simulink model "ame532Project1_GimbalDynamicsModel_2023a"  (R2023a)
settings: Solver=ode4  StartTime=0.0  StopTime=60  FixedStep=0.01  RelTol=1e-3
model workspace (MAT data in the model file):
  theta : Simulink.Parameter (value not decoded)
undefined symbols (not defined in the file): a0_s2, a0_s3, a0_s4, a0_s5, AR_s2, AR_s3, AR_s4, AR_s5, area_s2, area_s3, area_s4, area_s5, c_s2, c_s3, c_s4, c_s5, CD0_s2, CD0_s3, CD0_s4, CD0_s5, CDa_s2, CDa_s3, CDa_s4, CDa_s5, CL0_s2, CL0_s3, CL0_s4, CL0_s5, CM0_s2, CM0_s3, CM0_s4, CM0_s5, CMa_s2, CMa_s3, CMa_s4, CMa_s5, e_s2, e_s3, e_s4, e_s5, earthRadius, elevator_sA, i_s2, i_s3, i_s4, i_s5, Jxx, Jxy, Jxz, Jyx, Jyy, Jyz, Jzx, Jzy, Jzz, leftaileron_sA, LL, MM, n_s2, n_s3 ... (+12)
libraries: simulink_extras x35, matrix_library x23, aerolibutil x7, aerolibfltsims x4, vrlib x3, aerolibtransform2 x2, slpidlib x2, simulink x2, sharedutil x1
(part 2 of 4)

== system ame532Project1_GimbalDynamicsModel_2023a/Gimbal Aircraft dynamic sim/measurement subsystem ==
  velocity in body frame : Inport
  Asin : Trigonometry  Operator=asin
  Atan2 : Trigonometry  Operator=atan2
  Demux : Demux  Outputs=3
  Demux1 : Demux  Outputs=3
  Display : Display
  Divide : Product  Inputs=*/  RndMeth=Zero  SaturateOnIntegerOverflow=on
  MATLAB Function : MATLAB Function  TreatAsAtomicUnit=on
  Mux : Mux  Inputs=3
  Radians to Degrees{,1..3} (4 alike) : simulink_extras/Transformations/Radians to Degrees
  v_inf alpha beta : Scope  NumInputPorts=3
  total speed : Outport
  alpha (AoA) : Outport  Port=2
  beta (side slip) : Outport  Port=3
  wires:
  MATLAB Function/1(magnitude) -> Divide/2, Mux/1, total speed/1, v_inf alpha beta/1
  velocity in body frame/1 -> MATLAB Function/1(velocity), Demux1/1, Demux/1
  Demux/3 -> Atan2/1
  Demux/1 -> Atan2/2
  Atan2/1 -> alpha (AoA)/1, Radians to Degrees2/1, Radians to Degrees/1
  Demux1/2 -> Divide/1
  Divide/1 -> Asin/1
  Asin/1 -> beta (side slip)/1, Radians to Degrees3/1, Radians to Degrees1/1
  Mux/1 -> Display/1
  Radians to Degrees/1 -> Mux/2
  Radians to Degrees1/1 -> Mux/3
  Radians to Degrees2/1 -> v_inf alpha beta/2
  Radians to Degrees3/1 -> v_inf alpha beta/3

== system ame532Project1_GimbalDynamicsModel_2023a/Gimbal Aircraft dynamic sim/rotational dynamics ==
  note: body rate acceleration
  J_matrix : Inport
  Initial w : Inport  Port=2
  moment in body : Inport  Port=3
  Cross Product : matrix_library/Cross Product
  Display4 : Display
  Display5 : Display
  Display6 : Display
  Invert 3x3 Matrix : aerolibutil/Invert  3x3 Matrix
  Matrix Multiply4 : Product  Multiplication=Matrix(*)
  Matrix Multiply5 : Product  Multiplication=Matrix(*)
  Sum : Sum  Inputs=|+-
  body rate : Integrator  InitialConditionSource=external  InitialCondition=[0 0 0]'
  omega_b : Outport
  wires:
  Cross Product/1 -> Sum/2, Display6/1
  Sum/1 -> Matrix Multiply4/2
  J_matrix/1 -> Matrix Multiply5/1, Invert 3x3 Matrix/1
  body rate/1 -> omega_b/1, Matrix Multiply5/2, Cross Product/1
  Matrix Multiply4/1 -> Display5/1, body rate/1
  Invert 3x3 Matrix/1 -> Matrix Multiply4/1, Display4/1
  Matrix Multiply5/1 -> Cross Product/2
  Initial w/1 -> body rate/2
  moment in body/1 -> Sum/1

== system ame532Project1_GimbalDynamicsModel_2023a/Gimbal Aircraft dynamic sim/translational dynamics ==
  note: counter gravity before needs to be accounted by a DCM
  note: velocity in body frame
  note: acceleration in body frame
  p : Inport
  q : Inport  Port=2
  r : Inport  Port=3
  ZYXDCM : Inport  Port=4
  external forces : Inport  Port=5
  intial velocity : Inport  Port=6
  Display{,1..4,8..9} (7 alike) : Display
  Integrator5 : Integrator  InitialConditionSource=external
  MATLAB Function10 : MATLAB Function  TreatAsAtomicUnit=on
  Manual Switch : ManualSwitch
  Matrix Multiply6 : Product  Multiplication=Matrix(*)
  Matrix Multiply7 : Product  Multiplication=Matrix(*)
  Scope : Scope
  Sum : Sum  Inputs=|++-
  gravity in N_frame : Constant  Value=[0 0 9.81]'
  gravity in N_frame1 : Constant  Value=[0 0 0]'
  weight : Gain  Gain=1/0.48
  velocity in body frame : Outport
  wires:
  MATLAB Function10/1(Cross_Product_Matrix) -> Matrix Multiply7/1, Display8/1
  Integrator5/1 -> velocity in body frame/1, Display1/1, Matrix Multiply7/2
  Sum/1 -> Display3/1, Scope/1, Integrator5/1
  Matrix Multiply6/1 -> Sum/2, Display2/1
  Matrix Multiply7/1 -> Sum/3, Display9/1
  ZYXDCM/1 -> Display/1, Matrix Multiply6/1
  q/1 -> MATLAB Function10/2(q)
  p/1 -> MATLAB Function10/1(p)
  r/1 -> MATLAB Function10/3(r)
  intial velocity/1 -> Integrator5/2
  external forces/1 -> weight/1
  weight/1 -> Sum/1, Display4/1
  gravity in N_frame1/1 -> Manual Switch/2
  gravity in N_frame/1 -> Manual Switch/1
  Manual Switch/1 -> Matrix Multiply6/2

== system ame532Project1_GimbalDynamicsModel_2023a/Gimbal system/Controller  ==
  GA_Desired : Inport
  GA_True : Inport  Port=2
  Inport : Inport  Port=3
  J_Gimbal : Inport  Port=4
  Constant1 : Constant  Commented=on  Value=2
  Demux : Demux  Commented=on  Outputs=3
  Demux1 : Demux  Commented=on  Outputs=3
  Demux2 : Demux  Outputs=3
  Derivative : Derivative  Commented=on
  Derivative1 : Derivative  Commented=on
  Divide : Product  Commented=on  Inputs=*/
  Mux : Mux  Inputs=3
  PID Controller : slpidlib/PID Controller  Controller=PID  Form=Parallel  TimeDomain=Continuous-time  UseExternalTs=off  SampleTime=-1  IntegratorMethod=Forward Euler  FilterMethod=Forward Euler  ControllerParametersSource=internal  P=0.00204661863973543  I=7.76312130056365e-05  UseKiTs=off  D=0.0129825008664916  N=2.05306665016805  UseFilter=on  TunerSelectOption=Transfer Function Based (PID Tuner App)  InitialConditionSource=internal  InitialConditionForIntegrator=0  InitialConditionForFilter=0  DifferentiatorICPrevScaledInput=0  ExternalReset=none  TrackingMode=off  Kt=1  LimitOutput=off  SatLimitsSource=internal  UpperSaturationLimit=inf  LowerSaturationLimit=-inf  LinearizeAsGain=on  AntiWindupMode=none  Kb=1  LimitIntegrator=off  UpperIntegratorSaturationLimit=inf  LowerIntegratorSaturationLimit=-inf  POutMin=[]  POutMax=[]  IOutMin=[]  IOutMax=[]  DOutMin=[]  DOutMax=[]  NOutMin=[]  NOutMax=[]  SumOutMin=[]  SumOutMax=[]  SaturationOutMin=[]  SaturationOutMax=[]  PParamMin=[]  PParamMax=[]  IParamMin=[]  IParamMax=[]  DParamMin=[]  DParamMax=[]  NParamMin=[]  NParamMax=[]  KbParamMin=[]  KbParamMax=[]  KtParamMin=[]  KtParamMax=[]  KbOutMin=[]  KbOutMax=[]  KtOutMin=[]  KtOutMax=[]  IntegratorOutMin=[]  IntegratorOutMax=[]  FilterOutMin=[]  FilterOutMax=[]  SumI1OutMin=[]  SumI1OutMax=[]  SumI2OutMin=[]  SumI2OutMax=[]  SumI3OutMin=[]  SumI3OutMax=[]  SumI4OutMin=[]  SumI4OutMax=[]  SumDOutMin=[]  SumDOutMax=[]  DifferentiatorOutMin=[]  DifferentiatorOutMax=[]  FilterDiffOutCoefMin=[]  FilterDiffOutCoefMax=[]  ReciprocalOutMin=[]  ReciprocalOutMax=[]  SumDenOutMin=[]  SumDenOutMax=[]  SumNumOutMin=[]  SumNumOutMax=[]  DivideOutMin=[]  DivideOutMax=[]  UdiffTsProdOutMin=[]  UdiffTsProdOutMax=[]  NTsProdOutMin=[]  NTsProdOutMax=[]  UintegralTsProdOutMin=[]  UintegralTsProdOutMax=[]  UngainTsProdOutMin=[]  UngainTsProdOutMax=[]  ClampingZeroOutDataTypeStr=Inherit: Inherit via back propagation  ClampingZeroOutMin=[]  ClampingZeroOutMax=[]  FilterDenConstantOutDataTypeStr=Inherit: Inherit via back propagation  FilterDenConstantOutMin=[]  FilterDenConstantOutMax=[]  PCopyOutDataTypeStr=Inherit: Inherit via back propagation  PCopyOutMin=[]  PCopyOutMax=[]  NCopyOutDataTypeStr=Inherit: Inherit via back propagation  NCopyOutMin=[]  NCopyOutMax=[]  IntegratorContinuousStateAttributes=''  IntegratorStateMustResolveToSignalObject=off  IntegratorRTWStateStorageClass=Auto  FilterContinuousStateAttributes=''  FilterStateMustResolveToSignalObject=off  FilterRTWStateStorageClass=Auto  ParallelPVariant=InternalParameters  IdealPVariant=Disabled  IVariant=InternalParameters  DVariant=InternalParameters  IntegratorVariant=Continuous  SatVariant=Disabled  AWVariant=Passthrough  PCopyVariant=Disabled  TRVariant=Disabled  FdbkBlocksVariant=Forward  IdealPFdbkVariant=Disabled  SatFdbkVariant=Disabled  DerivativeFilterVariant=ContFilter  NVariant=InternalParameters  NCopyVariant=Disabled  FilterICVariant=InternalICsFilter  IntegratorICVariant=InternalICs  ExternalResetVariant=Disabled  TRSumVariant=Passthrough  SumFdbkVariant=Disabled  SumVariant=Sum_PID  TsampFilterVariant=InternalTs  TsampNgainVariant=Passthrough  TsampIntegralVariant=Disabled_SignalSpec  ExternalSaturationOutDataTypeStr=Inherit: Same as second input
  PID Controller1 : slpidlib/PID Controller  Controller=PID  Form=Parallel  TimeDomain=Continuous-time  UseExternalTs=off  SampleTime=-1  IntegratorMethod=Forward Euler  FilterMethod=Forward Euler  ControllerParametersSource=internal  P=-0.109538604051299  I=-0.0257010089513843  UseKiTs=off  D=-0.114637714712046  N=27.3346026399604  UseFilter=on  TunerSelectOption=Transfer Function Based (PID Tuner App)  InitialConditionSource=internal  InitialConditionForIntegrator=0  InitialConditionForFilter=0  DifferentiatorICPrevScaledInput=0  ExternalReset=none  TrackingMode=off  Kt=1  LimitOutput=off  SatLimitsSource=internal  UpperSaturationLimit=inf  LowerSaturationLimit=-inf  LinearizeAsGain=on  AntiWindupMode=none  Kb=1  LimitIntegrator=off  UpperIntegratorSaturationLimit=inf  LowerIntegratorSaturationLimit=-inf  POutMin=[]  POutMax=[]  IOutMin=[]  IOutMax=[]  DOutMin=[]  DOutMax=[]  NOutMin=[]  NOutMax=[]  SumOutMin=[]  SumOutMax=[]  SaturationOutMin=[]  SaturationOutMax=[]  PParamMin=[]  PParamMax=[]  IParamMin=[]  IParamMax=[]  DParamMin=[]  DParamMax=[]  NParamMin=[]  NParamMax=[]  KbParamMin=[]  KbParamMax=[]  KtParamMin=[]  KtParamMax=[]  KbOutMin=[]  KbOutMax=[]  KtOutMin=[]  KtOutMax=[]  IntegratorOutMin=[]  IntegratorOutMax=[]  FilterOutMin=[]  FilterOutMax=[]  SumI1OutMin=[]  SumI1OutMax=[]  SumI2OutMin=[]  SumI2OutMax=[]  SumI3OutMin=[]  SumI3OutMax=[]  SumI4OutMin=[]  SumI4OutMax=[]  SumDOutMin=[]  SumDOutMax=[]  DifferentiatorOutMin=[]  DifferentiatorOutMax=[]  FilterDiffOutCoefMin=[]  FilterDiffOutCoefMax=[]  ReciprocalOutMin=[]  ReciprocalOutMax=[]  SumDenOutMin=[]  SumDenOutMax=[]  SumNumOutMin=[]  SumNumOutMax=[]  DivideOutMin=[]  DivideOutMax=[]  UdiffTsProdOutMin=[]  UdiffTsProdOutMax=[]  NTsProdOutMin=[]  NTsProdOutMax=[]  UintegralTsProdOutMin=[]  UintegralTsProdOutMax=[]  UngainTsProdOutMin=[]  UngainTsProdOutMax=[]  ClampingZeroOutDataTypeStr=Inherit: Inherit via back propagation  ClampingZeroOutMin=[]  ClampingZeroOutMax=[]  FilterDenConstantOutDataTypeStr=Inherit: Inherit via back propagation  FilterDenConstantOutMin=[]  FilterDenConstantOutMax=[]  PCopyOutDataTypeStr=Inherit: Inherit via back propagation  PCopyOutMin=[]  PCopyOutMax=[]  NCopyOutDataTypeStr=Inherit: Inherit via back propagation  NCopyOutMin=[]  NCopyOutMax=[]  IntegratorContinuousStateAttributes=''  IntegratorStateMustResolveToSignalObject=off  IntegratorRTWStateStorageClass=Auto  FilterContinuousStateAttributes=''  FilterStateMustResolveToSignalObject=off  FilterRTWStateStorageClass=Auto  ParallelPVariant=InternalParameters  IdealPVariant=Disabled  IVariant=InternalParameters  DVariant=InternalParameters  IntegratorVariant=Continuous  SatVariant=Disabled  AWVariant=Passthrough  PCopyVariant=Disabled  TRVariant=Disabled  FdbkBlocksVariant=Forward  IdealPFdbkVariant=Disabled  SatFdbkVariant=Disabled  DerivativeFilterVariant=ContFilter  NVariant=InternalParameters  NCopyVariant=Disabled  FilterICVariant=InternalICsFilter  IntegratorICVariant=InternalICs  ExternalResetVariant=Disabled  TRSumVariant=Passthrough  SumFdbkVariant=Disabled  SumVariant=Sum_PID  TsampFilterVariant=InternalTs  TsampNgainVariant=Passthrough  TsampIntegralVariant=Disabled_SignalSpec  ExternalSaturationOutDataTypeStr=Inherit: Same as second input
  Product : Product  Commented=on
  Product1 : Product  Commented=on
  Product2 : Product  Multiplication=Matrix(*)
  Scope : Scope
  Scope1 : Scope
  Square : Math  Commented=on  Operator=square
  Subtract : Sum  Inputs=+-
  Subtract1 : Sum  Commented=on  Inputs=+-
  time : Constant  Commented=on  Value=5
  Torque_Cmd : Outport
  wires:
  GA_Desired/1 -> Subtract/1
  GA_True/1 -> Subtract/2
  Derivative/1 -> Derivative1/1
  Derivative1/1 -> Demux1/1
  Inport/1 -> Product/1
  time/1 -> Product/2, Square/1
  Product/1 -> Subtract1/2
  Subtract1/1 -> Product1/1
  Constant1/1 -> Product1/2
  Product1/1 -> Divide/1
  Square/1 -> Divide/2
  Product2/1 -> Scope1/1
  Subtract/1 -> Demux2/1
  Demux2/2 -> PID Controller/1
  Demux2/3 -> PID Controller1/1
  PID Controller/1 -> Mux/2
  PID Controller1/1 -> Mux/3
  Demux2/1 -> Mux/1
  Mux/1 -> Torque_Cmd/1

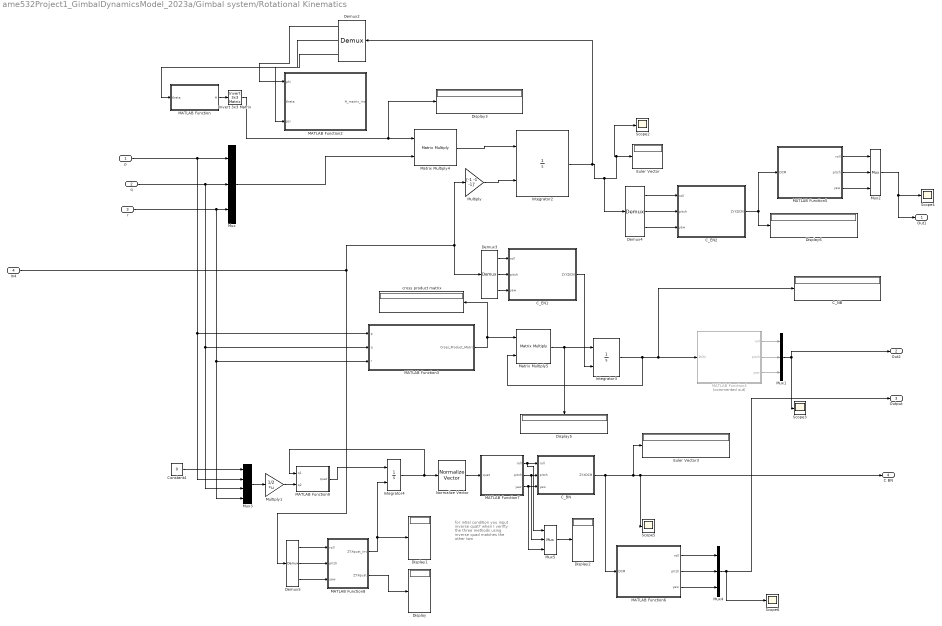
== system ame532Project1_GimbalDynamicsModel_2023a/Gimbal system/Rotational Kinematics ==
  note: for intial condition you input inverse quat?
      | when I verifty the three methods using inverse quad matches the other two
  p : Inport
  q : Inport  Port=2
  r : Inport  Port=3
  In4 : Inport  Port=4
  C_BN : MATLAB Function  TreatAsAtomicUnit=on
  C_EN1 : MATLAB Function  TreatAsAtomicUnit=on
  C_EN2 : MATLAB Function  TreatAsAtomicUnit=on
  C_NB : Display
  Constant4 : Constant  Value=0
  Demux{2..5} (4 alike) : Demux  Outputs=3
  Display{,1..3,5..6} (6 alike) : Display
  Euler Vector : Display
  Euler Vector3 : Display
  Integrator2 : Integrator  InitialConditionSource=external
  Integrator3 : Integrator  InitialConditionSource=external
  Integrator4 : Integrator  InitialConditionSource=external  InitialCondition=[1 0 0 0]'
  Invert 3x3 Matrix : aerolibutil/Invert  3x3 Matrix
  MATLAB Function : MATLAB Function  TreatAsAtomicUnit=on
  MATLAB Function2 : MATLAB Function  TreatAsAtomicUnit=on
  MATLAB Function3 : MATLAB Function  TreatAsAtomicUnit=on
  MATLAB Function4 : MATLAB Function  Commented=on  TreatAsAtomicUnit=on
  MATLAB Function5 : MATLAB Function  TreatAsAtomicUnit=on
  MATLAB Function6 : MATLAB Function  TreatAsAtomicUnit=on
  MATLAB Function7 : MATLAB Function  TreatAsAtomicUnit=on
  MATLAB Function8 : MATLAB Function  TreatAsAtomicUnit=on
  MATLAB Function9 : MATLAB Function  TreatAsAtomicUnit=on
  Matrix Multiply4 : Product  Multiplication=Matrix(*)
  Matrix Multiply5 : Product  Multiplication=Matrix(*)
  Multiply : Gain  Gain=[-1 -1 -1]'
  Multiply1 : Gain  Gain=1/2  Multiplication=Matrix(K*u)
  Mux{,1..2,4..5} (5 alike) : Mux  Inputs=3
  Mux3 : Mux
  Normalize Vector : vrlib/Utilities/Normalize Vector  maxzero=0
  Scope{2..6} (5 alike) : Scope
  cross product matrix : Display
  Out1 : Outport
  Out2 : Outport  Port=2
  Output : Outport  Port=3
  C BN : Outport  Port=4
  wires:
  Matrix Multiply4/1 -> Integrator2/1
  In4/1 -> Multiply/1, Demux3/1, Demux5/1
  MATLAB Function4/3(yaw) -> Mux1/3
  Integrator2/1 -> Scope2/1, Euler Vector/1, Demux4/1, Demux2/1
  MATLAB Function6/2(pitch) -> Mux4/2
  r/1 -> Mux3/4, MATLAB Function3/3(r), Mux/3
  Matrix Multiply5/1 -> Display5/1, Integrator3/1
  Mux/1 -> Matrix Multiply4/2
  q/1 -> Mux3/3, MATLAB Function3/2(q), Mux/2
  C_BN/1(ZYXDCM) -> MATLAB Function6/1(DCM), C BN/1, Scope5/1, Euler Vector3/1
  C_EN1/1(ZYXDCM) -> Integrator3/2
  MATLAB Function5/2(pitch) -> Mux2/2
  Mux1/1 -> Out2/1, Scope3/1
  MATLAB Function4/1(roll) -> Mux1/1
  Demux2/2 -> MATLAB Function/1(theta)
  Demux4/3 -> C_EN2/3(yaw)
  MATLAB Function4/2(pitch) -> Mux1/2
  Demux2/3 -> MATLAB Function2/3(psi)
  Demux2/1 -> MATLAB Function2/1(phi)
  Demux5/1 -> MATLAB Function8/1(roll)
  Demux3/1 -> C_EN1/1(roll)
  Demux5/2 -> MATLAB Function8/2(pitch)
  Demux4/1 -> C_EN2/1(roll)
  Demux3/3 -> C_EN1/3(yaw)
  Multiply/1 -> Integrator2/2
  C_EN2/1(ZYXDCM) -> Display6/1, MATLAB Function5/1(DCM)
  Normalize Vector/1 -> MATLAB Function7/1(quat)
  MATLAB Function9/1(quat) -> Integrator4/1
  Integrator3/1 -> Matrix Multiply5/2, MATLAB Function4/1(DCM), C_NB/1
  p/1 -> Mux3/2, MATLAB Function3/1(p), Mux/1
  Integrator4/1 -> Normalize Vector/1, MATLAB Function9/1(q1)
  MATLAB Function7/3(yaw) -> Mux5/3, C_BN/3(yaw)
  Mux2/1 -> Out1/1, Scope4/1
  MATLAB Function5/3(yaw) -> Mux2/3
  Constant4/1 -> Mux3/1
  Mux3/1 -> Multiply1/1
  Mux4/1 -> Output/1, Scope6/1
  MATLAB Function7/1(roll) -> Mux5/1, C_BN/1(roll)
  MATLAB Function5/1(roll) -> Mux2/1
  Demux5/3 -> MATLAB Function8/3(yaw)
  MATLAB Function6/1(roll) -> Mux4/1
  MATLAB Function6/3(yaw) -> Mux4/3
  Multiply1/1 -> MATLAB Function9/2(q2)
  MATLAB Function3/1(Cross_Product_Matrix) -> Matrix Multiply5/1, cross product matrix/1
  Demux4/2 -> C_EN2/2(pitch)
  Demux3/2 -> C_EN1/2(pitch)
  MATLAB Function7/2(pitch) -> Mux5/2, C_BN/2(pitch)
  MATLAB Function8/1(ZYXquat_inv) -> Integrator4/2, Display1/1
  MATLAB Function8/2(ZYXquat) -> Display/1
  Mux5/1 -> Display2/1
  MATLAB Function/1(H) -> Invert 3x3 Matrix/1
  Invert 3x3 Matrix/1 -> Display3/1, Matrix Multiply4/1

== system ame532Project1_GimbalDynamicsModel_2023a/Gimbal system/rotational dynamics gimbal ==
  note: body acceleration
  J_matrix : Inport
  Initial w : Inport  Port=2
  Tcmd : Inport  Port=3
  Cross Product : matrix_library/Cross Product
  Display4 : Display
  Display5 : Display
  Display6 : Display
  Invert 3x3 Matrix : aerolibutil/Invert  3x3 Matrix
  Matrix Multiply4 : Product  Multiplication=Matrix(*)
  Matrix Multiply5 : Product  Multiplication=Matrix(*)
  Sum : Sum  Inputs=|+-
  body rate : Integrator  InitialConditionSource=external  InitialCondition=[0 0 0]'
  w_b : Outport
  Outport : Outport  Port=2
  wires:
  Cross Product/1 -> Sum/2, Display6/1
  Sum/1 -> Matrix Multiply4/2
  J_matrix/1 -> Matrix Multiply5/1, Invert 3x3 Matrix/1
  body rate/1 -> w_b/1, Matrix Multiply5/2, Cross Product/1
  Matrix Multiply4/1 -> Display5/1, Outport/1, body rate/1
  Matrix Multiply5/1 -> Cross Product/2
  Initial w/1 -> body rate/2
  Tcmd/1 -> Sum/1
  Invert 3x3 Matrix/1 -> Display4/1, Matrix Multiply4/1

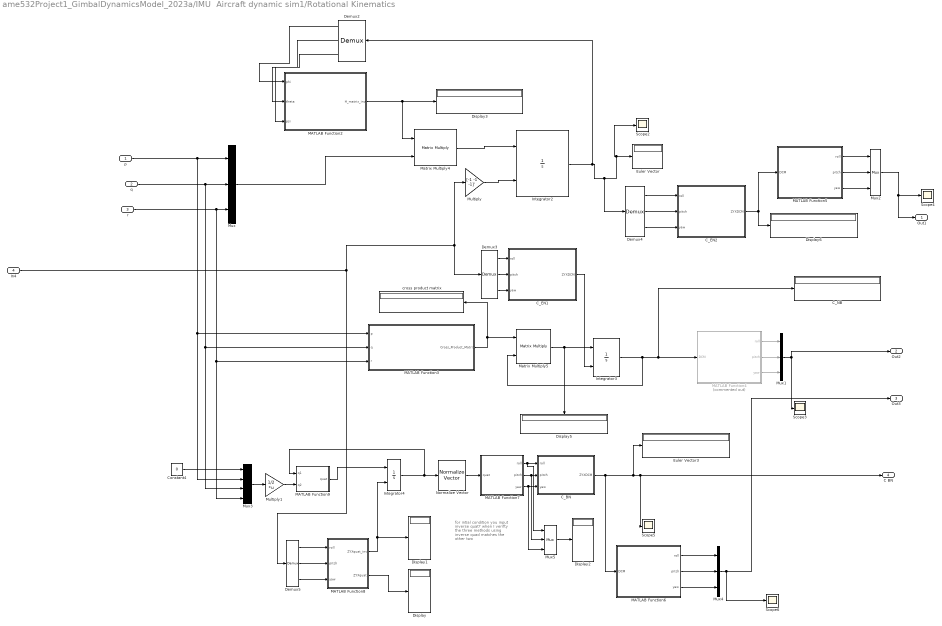
== system ame532Project1_GimbalDynamicsModel_2023a/IMU  Aircraft dynamic sim1/Rotational Kinematics ==
  note: for intial condition you input inverse quat?
      | when I verifty the three methods using inverse quad matches the other two
  p : Inport
  q : Inport  Port=2
  r : Inport  Port=3
  In4 : Inport  Port=4
  C_BN : MATLAB Function  TreatAsAtomicUnit=on
  C_EN1 : MATLAB Function  TreatAsAtomicUnit=on
  C_EN2 : MATLAB Function  TreatAsAtomicUnit=on
  C_NB : Display
  Constant4 : Constant  Value=0
  Demux{2..5} (4 alike) : Demux  Outputs=3
  Display{,1..3,5..6} (6 alike) : Display
  Euler Vector : Display
  Euler Vector3 : Display
  Integrator2 : Integrator  InitialConditionSource=external
  Integrator3 : Integrator  InitialConditionSource=external
  Integrator4 : Integrator  InitialConditionSource=external  InitialCondition=[1 0 0 0]'
  MATLAB Function2 : MATLAB Function  TreatAsAtomicUnit=on
  MATLAB Function3 : MATLAB Function  TreatAsAtomicUnit=on
  MATLAB Function4 : MATLAB Function  Commented=on  TreatAsAtomicUnit=on
  MATLAB Function5 : MATLAB Function  TreatAsAtomicUnit=on
  MATLAB Function6 : MATLAB Function  TreatAsAtomicUnit=on
  MATLAB Function7 : MATLAB Function  TreatAsAtomicUnit=on
  MATLAB Function8 : MATLAB Function  TreatAsAtomicUnit=on
  MATLAB Function9 : MATLAB Function  TreatAsAtomicUnit=on
  Matrix Multiply4 : Product  Multiplication=Matrix(*)
  Matrix Multiply5 : Product  Multiplication=Matrix(*)
  Multiply : Gain  Gain=[-1 -1 -1]'
  Multiply1 : Gain  Gain=1/2  Multiplication=Matrix(K*u)
  Mux{,1..2,4..5} (5 alike) : Mux  Inputs=3
  Mux3 : Mux
  Normalize Vector : vrlib/Utilities/Normalize Vector  maxzero=0
  Scope{2..6} (5 alike) : Scope
  cross product matrix : Display
  Out1 : Outport
  Out2 : Outport  Port=2
  Out3 : Outport  Port=3
  C BN : Outport  Port=4
  wires:
  Matrix Multiply4/1 -> Integrator2/1
  In4/1 -> Multiply/1, Demux3/1, Demux5/1
  MATLAB Function4/3(yaw) -> Mux1/3
  Integrator2/1 -> Scope2/1, Euler Vector/1, Demux4/1, Demux2/1
  MATLAB Function2/1(H_matrix_inv) -> Display3/1, Matrix Multiply4/1
  MATLAB Function6/2(pitch) -> Mux4/2
  r/1 -> Mux3/4, MATLAB Function3/3(r), Mux/3
  Matrix Multiply5/1 -> Display5/1, Integrator3/1
  Mux/1 -> Matrix Multiply4/2
  q/1 -> Mux3/3, MATLAB Function3/2(q), Mux/2
  C_BN/1(ZYXDCM) -> MATLAB Function6/1(DCM), C BN/1, Scope5/1, Euler Vector3/1
  C_EN1/1(ZYXDCM) -> Integrator3/2
  MATLAB Function5/2(pitch) -> Mux2/2
  Mux1/1 -> Out2/1, Scope3/1
  MATLAB Function4/1(roll) -> Mux1/1
  Demux2/2 -> MATLAB Function2/2(theta)
  Demux4/3 -> C_EN2/3(yaw)
  MATLAB Function4/2(pitch) -> Mux1/2
  Demux2/3 -> MATLAB Function2/3(psi)
  Demux2/1 -> MATLAB Function2/1(phi)
  Demux5/1 -> MATLAB Function8/1(roll)
  Demux3/1 -> C_EN1/1(roll)
  Demux5/2 -> MATLAB Function8/2(pitch)
  Demux4/1 -> C_EN2/1(roll)
  Demux3/3 -> C_EN1/3(yaw)
  Multiply/1 -> Integrator2/2
  C_EN2/1(ZYXDCM) -> Display6/1, MATLAB Function5/1(DCM)
  Normalize Vector/1 -> MATLAB Function7/1(quat)
  MATLAB Function9/1(quat) -> Integrator4/1
  Integrator3/1 -> Matrix Multiply5/2, MATLAB Function4/1(DCM), C_NB/1
  p/1 -> Mux3/2, MATLAB Function3/1(p), Mux/1
  Integrator4/1 -> Normalize Vector/1, MATLAB Function9/1(q1)
  MATLAB Function7/3(yaw) -> Mux5/3, C_BN/3(yaw)
  Mux2/1 -> Out1/1, Scope4/1
  MATLAB Function5/3(yaw) -> Mux2/3
  Constant4/1 -> Mux3/1
  Mux3/1 -> Multiply1/1
  Mux4/1 -> Out3/1, Scope6/1
  MATLAB Function7/1(roll) -> Mux5/1, C_BN/1(roll)
  MATLAB Function5/1(roll) -> Mux2/1
  Demux5/3 -> MATLAB Function8/3(yaw)
  MATLAB Function6/1(roll) -> Mux4/1
  MATLAB Function6/3(yaw) -> Mux4/3
  Multiply1/1 -> MATLAB Function9/2(q2)
  MATLAB Function3/1(Cross_Product_Matrix) -> Matrix Multiply5/1, cross product matrix/1
  Demux4/2 -> C_EN2/2(pitch)
  Demux3/2 -> C_EN1/2(pitch)
  MATLAB Function7/2(pitch) -> Mux5/2, C_BN/2(pitch)
  MATLAB Function8/1(ZYXquat_inv) -> Integrator4/2, Display1/1
  MATLAB Function8/2(ZYXquat) -> Display/1
  Mux5/1 -> Display2/1

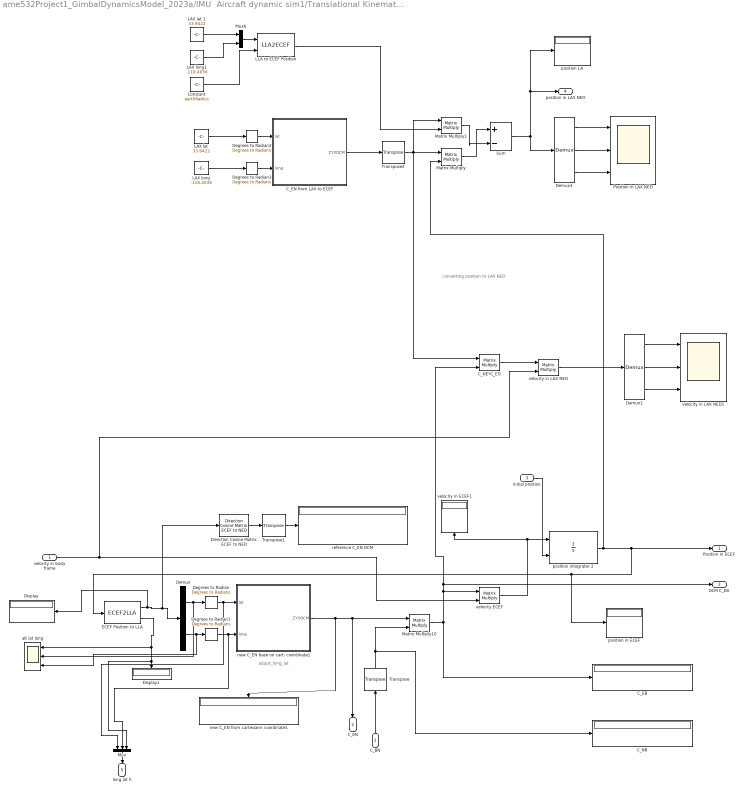
== system ame532Project1_GimbalDynamicsModel_2023a/IMU  Aircraft dynamic sim1/Translational Kinematics ==
  note: converting position to LAX NED
  note: adjust_long_lat
  velocity in body frame : Inport
  C_BN : Inport  Port=2
  initial position : Inport  Port=3
  C_EB : Display
  C_EN from LAX to ECEF : MATLAB Function  TreatAsAtomicUnit=on
  C_NB : Display
  C_NE*C_EO : Product  Multiplication=Matrix(*)
  Constant : Constant  Value=earthRadius
  Degrees to Radian{,1..3} (4 alike) : simulink_extras/Transformations/Degrees to Radians
  Demux : Demux  Outputs=2
  Demux1 : Demux  Outputs=3
  Demux3 : Demux  Outputs=3
  Direction Cosine Matrix ECEF to NED : aerolibtransform2/Direction Cosine Matrix ECEF to NED
  Display : Display
  Display1 : Display
  ECEF Position to LLA : ECEF2LLA  ptype=Custom  R=earthRadius
  "LAX lat " : Constant  Value=33.9422
  LAX lat 1 : Constant  Value=33.9422
  LAX long : Constant  Value=-118.4036
  LAX long1 : Constant  Value=-118.4036
  LLA to ECEF Position : LLA2ECEF
  Matrix Multiply : Product  Multiplication=Matrix(*)
  Matrix Multiply1 : Product  Multiplication=Matrix(*)
  Matrix Multiply10 : Product  Multiplication=Matrix(*)
  Mux : Mux  Inputs=3
  Mux6 : Mux  Inputs=2
  Position in LAX NED : Scope  NumInputPorts=3
  Sum : Sum  Inputs=|+-
  Transpose : matrix_library/Transpose
  Transpose1 : matrix_library/Transpose
  Transpose2 : matrix_library/Transpose
  alt lat long : Scope  NumInputPorts=3
  new C_EN base on cart. coordinate1 : MATLAB Function  TreatAsAtomicUnit=on
  new C_EN from cartesiann coordinate1 : Display
  "position LA " : Display
  position in ECEF : Display
  position integrator 2 : Integrator  InitialConditionSource=external  InitialCondition=[6378100,0,0]'
  reference C_EN DCM : Display
  velocity ECEF : Product  Multiplication=Matrix(*)
  velocity in ECEF1 : Display
  velocity in LAX NED : Product  Multiplication=Matrix(*)
  velocity in LAX NED1 : Scope  NumInputPorts=3
  Position in ECEF : Outport
  C_EN : Outport  Port=2
  DCM C_EB : Outport  Port=3
  position in LAX NED : Outport  Port=4
  long lat h : Outport  Port=5
  wires:
  initial position/1 -> position integrator 2/2
  new C_EN base on cart. coordinate1/1(ZYXDCM) -> new C_EN from cartesiann coordinate1/1, C_EN/1, Matrix Multiply10/1
  Matrix Multiply10/1 -> C_EB/1, DCM C_EB/1, C_NE*C_EO/2, velocity ECEF/1
  velocity ECEF/1 -> position integrator 2/1, velocity in ECEF1/1
  velocity in body frame/1 -> velocity in LAX NED/2, velocity ECEF/2
  C_BN/1 -> Transpose/1
  ECEF Position to LLA/1 -> Direction Cosine Matrix ECEF to NED/1, Demux/1, Display/1
  ECEF Position to LLA/2 -> alt lat long/1, Mux/3, Display1/1
  Demux/1 -> Degrees to Radian/1, alt lat long/2
  Demux/2 -> alt lat long/3, Degrees to Radian1/1
  Degrees to Radian/1 -> Mux/1, new C_EN base on cart. coordinate1/1(lat)
  Degrees to Radian1/1 -> Mux/2, new C_EN base on cart. coordinate1/2(long)
  Transpose/1 -> C_NB/1, Matrix Multiply10/2
  Direction Cosine Matrix ECEF to NED/1 -> Transpose1/1
  Transpose1/1 -> reference C_EN DCM/1
  Mux/1 -> long lat h/1
  "LAX lat "/1 -> Degrees to Radian2/1
  LAX long/1 -> Degrees to Radian3/1
  Degrees to Radian2/1 -> C_EN from LAX to ECEF/1(lat)
  Degrees to Radian3/1 -> C_EN from LAX to ECEF/2(long)
  C_EN from LAX to ECEF/1(ZYXDCM) -> Transpose2/1
  Demux3/2 -> Position in LAX NED/2
  Demux3/3 -> Position in LAX NED/3
  Demux3/1 -> Position in LAX NED/1
  Transpose2/1 -> C_NE*C_EO/1, Matrix Multiply1/1, Matrix Multiply/1
  LAX long1/1 -> Mux6/2
  LAX lat 1/1 -> Mux6/1
  Constant/1 -> LLA to ECEF Position/2
  Mux6/1 -> LLA to ECEF Position/1
  LLA to ECEF Position/1 -> Matrix Multiply1/2
  Matrix Multiply/1 -> Sum/1
  Matrix Multiply1/1 -> Sum/2
  Sum/1 -> "position LA "/1, position in LAX NED/1, Demux3/1
  position integrator 2/1 -> Position in ECEF/1, ECEF Position to LLA/1, position in ECEF/1, Matrix Multiply/2
  C_NE*C_EO/1 -> velocity in LAX NED/1
  Demux1/2 -> velocity in LAX NED1/2
  velocity in LAX NED/1 -> Demux1/1
  Demux1/3 -> velocity in LAX NED1/3
  Demux1/1 -> velocity in LAX NED1/1

== system ame532Project1_GimbalDynamicsModel_2023a/IMU  Aircraft dynamic sim1/Unused tranlational kinmatics ==
  In1 : Inport
  In2 : Inport  Port=2
  In3 : Inport  Port=3
  C_EN4 : MATLAB Function  TreatAsAtomicUnit=on
  DCM4 : Display
  Matrix Multiply8 : Product  Multiplication=Matrix(*)
  Matrix Multiply9 : Product  Multiplication=Matrix(*)
  Scope7 : Scope
  Transpose : matrix_library/Transpose
  pitch4 : Constant  Value=pi/2
  position integrator 1 : Integrator  InitialConditionSource=external  InitialCondition=[6378100,0,0]'
  position vector2 : Display
  roll4 : Constant  Value=0
  velocity in earth frame : Display
  yaw4 : Constant  Value=0
  wires:
  Matrix Multiply9/1 -> DCM4/1, Matrix Multiply8/1
  position integrator 1/1 -> Scope7/1, position vector2/1
  C_EN4/1(ZYXDCM) -> Matrix Multiply9/1
  Matrix Multiply8/1 -> velocity in earth frame/1, position integrator 1/1
  yaw4/1 -> C_EN4/3(yaw)
  pitch4/1 -> C_EN4/2(pitch)
  Transpose/1 -> Matrix Multiply9/2
  roll4/1 -> C_EN4/1(roll)
  In2/1 -> Matrix Multiply8/2
  In1/1 -> position integrator 1/2
  In3/1 -> Transpose/1

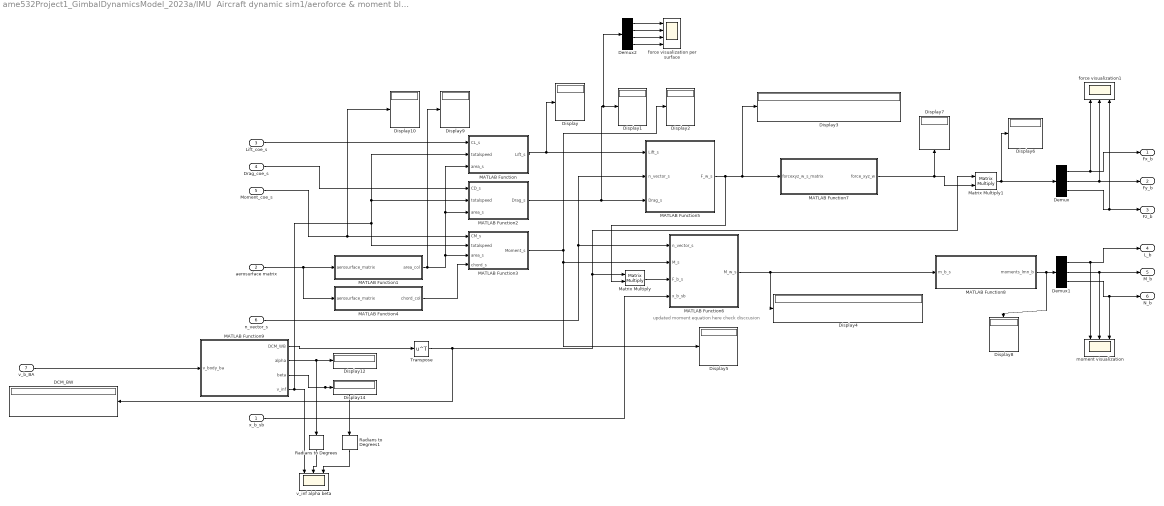
== system ame532Project1_GimbalDynamicsModel_2023a/IMU  Aircraft dynamic sim1/aeroforce & moment block ==
  note: updated moment equation here check disccusion
  x_b_sb : Inport
  aerosurface matrix : Inport  Port=2
  Lift_coe_s : Inport  Port=3
  Drag_coe_s : Inport  Port=4
  Moment_coe_s : Inport  Port=5
  n_vector_s : Inport  Port=6
  v_b_BA : Inport  Port=7
  DCM_BW : Display
  Demux : Demux  Outputs=3
  Demux1 : Demux  Outputs=3
  Demux2 : Demux
  Display{,1..10,12,14} (13 alike) : Display
  MATLAB Function : MATLAB Function  TreatAsAtomicUnit=on
  MATLAB Function1 : MATLAB Function  TreatAsAtomicUnit=on
  MATLAB Function2 : MATLAB Function  TreatAsAtomicUnit=on
  MATLAB Function3 : MATLAB Function  TreatAsAtomicUnit=on
  MATLAB Function4 : MATLAB Function  TreatAsAtomicUnit=on
  MATLAB Function5 : MATLAB Function  TreatAsAtomicUnit=on
  MATLAB Function6 : MATLAB Function  TreatAsAtomicUnit=on
  MATLAB Function7 : MATLAB Function  TreatAsAtomicUnit=on
  MATLAB Function8 : MATLAB Function  TreatAsAtomicUnit=on
  MATLAB Function9 : MATLAB Function  TreatAsAtomicUnit=on
  Matrix Multiply : Product  Multiplication=Matrix(*)
  Matrix Multiply1 : Product  Multiplication=Matrix(*)
  Radians to Degrees : simulink_extras/Transformations/Radians to Degrees
  Radians to Degrees1 : simulink_extras/Transformations/Radians to Degrees
  Transpose : Math  Operator=transpose
  force visualization per surface : Scope  NumInputPorts=4
  force visualization1 : Scope  NumInputPorts=3
  moment visualization : Scope  NumInputPorts=3
  v_inf alpha beta : Scope  NumInputPorts=3
  Fx_b : Outport
  Fy_b : Outport  Port=2
  Fz_b : Outport  Port=3
  L_b : Outport  Port=4
  M_b : Outport  Port=5
  N_b : Outport  Port=6
  wires:
  Lift_coe_s/1 -> MATLAB Function/1(CL_s)
  MATLAB Function9/4(v_inf) -> v_inf alpha beta/1, MATLAB Function2/2(totalspeed), MATLAB Function/2(totalspeed), MATLAB Function3/2(totalspeed)
  aerosurface matrix/1 -> MATLAB Function4/1(aerosurface_matrix), MATLAB Function1/1(aerosurface_matrix)
  MATLAB Function1/1(area_col) -> Display9/1, MATLAB Function2/3(area_s), MATLAB Function/3(area_s), MATLAB Function3/3(area_s)
  Drag_coe_s/1 -> MATLAB Function2/1(CD_s)
  Moment_coe_s/1 -> Display10/1, MATLAB Function3/1(CM_s)
  MATLAB Function4/1(chord_col) -> MATLAB Function3/4(chord_s)
  n_vector_s/1 -> MATLAB Function5/2(n_vector_s), MATLAB Function6/1(n_vector_s)
  MATLAB Function/1(Lift_s) -> Display/1, MATLAB Function5/1(Lift_s)
  MATLAB Function2/1(Drag_s) -> MATLAB Function5/3(Drag_s), Demux2/1, Display1/1
  MATLAB Function3/1(Moment_s) -> Display5/1, MATLAB Function6/2(M_s), Display2/1
  MATLAB Function6/1(M_w_s) -> Display4/1, MATLAB Function8/1(m_b_s)
  Matrix Multiply/1 -> MATLAB Function6/3(F_b_s)
  x_b_sb/1 -> MATLAB Function6/4(x_b_sb)
  MATLAB Function5/1(F_w_s) -> Matrix Multiply/2, Display3/1, MATLAB Function7/1(forcexyz_w_s_matrix)
  MATLAB Function7/1(force_xyz_w) -> Matrix Multiply1/2, Display7/1
  MATLAB Function8/1(moments_lmn_b) -> Demux1/1, Display8/1
  Matrix Multiply1/1 -> Demux/1, Display6/1
  MATLAB Function9/1(DCM_WB) -> Transpose/1
  v_b_BA/1 -> MATLAB Function9/1(v_body_ba)
  MATLAB Function9/2(alpha) -> Radians to Degrees/1, Display12/1
  MATLAB Function9/3(beta) -> Display14/1, Radians to Degrees1/1
  Demux1/1 -> L_b/1, moment visualization/1
  Demux1/2 -> M_b/1, moment visualization/2
  Demux1/3 -> moment visualization/3, N_b/1
  Demux/1 -> Fx_b/1, force visualization1/1
  Demux/2 -> Fy_b/1, force visualization1/2
  Demux/3 -> Fz_b/1, force visualization1/3
  Transpose/1 -> Matrix Multiply1/1, Matrix Multiply/1, DCM_BW/1
  Radians to Degrees/1 -> v_inf alpha beta/2
  Radians to Degrees1/1 -> v_inf alpha beta/3
  Demux2/4 -> force visualization per surface/4
  Demux2/3 -> force visualization per surface/3
  Demux2/2 -> force visualization per surface/2
  Demux2/1 -> force visualization per surface/1

== system ame532Project1_GimbalDynamicsModel_2023a/IMU  Aircraft dynamic sim1/aeroforce coefficient block ==
  note: next step is to create lift force, CD, CM
  aero surface property matrix : Inport
  real wind in N axes : Inport  Port=2
  velocity in bodyframe : Inport  Port=3
  C_BN : Inport  Port=4
  CD0 : Constant  Value=[0.01 0.01 0.01 0.01]'
  CD1 : Constant  Value=[0.9 0.9 0.8 0.8]'
  CD_a : Constant  Value=[1 1 1 1]'
  CL over time : Scope  NumInputPorts=4
  CL0 : Constant  Value=[0.05 0.05 0 0]'
  CM_0 : Constant  Value=[-0.05 -0.05 0 0]'
  CM_a : Constant  Value=[0 0 0 0]'
  Demux1 : Demux
  Demux5 : Demux
  Demux6 : Demux  Outputs=3
  Display{,1..3,5..7} (7 alike) : Display
  MATLAB Function : MATLAB Function  TreatAsAtomicUnit=on
  MATLAB Function1 : MATLAB Function  TreatAsAtomicUnit=on
  MATLAB Function2 : MATLAB Function  TreatAsAtomicUnit=on
  MATLAB Function3 : MATLAB Function  TreatAsAtomicUnit=on
  alpha : Scope  NumInputPorts=4
  alpha_0 : Constant  Value=[0.05 0.05 0 0]'
  calculatie alpha : MATLAB Function  TreatAsAtomicUnit=on
  extract matrix function : MATLAB Function  TreatAsAtomicUnit=on
  extract matrix function1 : MATLAB Function  TreatAsAtomicUnit=on
  i0 : Constant  Value=[0.05 0.05 0 0]'
  n vector(4 5 2 3 from left to right) : Constant  Value=[0 0 0 0;0 0 0 1;-1 -1 -1 0]
  velocity in body wrt air : Scope  NumInputPorts=3
  Lift coefficient_s : Outport
  Drag coefficient_s : Outport  Port=2
  Moment coefficient_s : Outport  Port=3
  n_vector_s : Outport  Port=4
  v_B_BA : Outport  Port=5
  wires:
  aero surface property matrix/1 -> extract matrix function1/1(aero_surface_matrix), extract matrix function/1(aero_surface_matrix)
  extract matrix function/1(AR_matrix) -> Display/1, MATLAB Function/1(AR_matrix)
  MATLAB Function/1(CL_a) -> MATLAB Function1/2(CL_a), Display1/1
  n vector(4 5 2 3 from left to right)/1 -> n_vector_s/1, calculatie alpha/3(n_vector)
  velocity in bodyframe/1 -> calculatie alpha/2(v_B)
  i0/1 -> calculatie alpha/1(i0)
  CL0/1 -> MATLAB Function1/1(CL0)
  Demux5/2 -> CL over time/2
  Demux5/1 -> CL over time/1
  Demux5/3 -> CL over time/3
  MATLAB Function1/1(CL_s) -> Demux5/1, Display3/1, Lift coefficient_s/1, MATLAB Function2/5(CL_s)
  Demux5/4 -> CL over time/4
  real wind in N axes/1 -> calculatie alpha/4(wind_w)
  extract matrix function1/1(AR_matrix) -> MATLAB Function2/7(AR)
  CD1/1 -> MATLAB Function2/6(e)
  alpha_0/1 -> MATLAB Function2/3(alpha_0)
  CD0/1 -> MATLAB Function2/1(CD_0)
  CD_a/1 -> MATLAB Function2/2(CD_a)
  MATLAB Function2/1(CD_s) -> Drag coefficient_s/1, Display6/1
  CM_0/1 -> MATLAB Function3/2(CM_0)
  CM_a/1 -> MATLAB Function3/3(CM_a)
  MATLAB Function3/1(CM_s) -> Moment coefficient_s/1, Display7/1
  C_BN/1 -> calculatie alpha/5(C_BN)
  calculatie alpha/2(v_B_BA) -> Demux6/1, Display5/1, v_B_BA/1
  Demux6/3 -> velocity in body wrt air/3
  Demux6/2 -> velocity in body wrt air/2
  Demux6/1 -> velocity in body wrt air/1
  Demux1/1 -> alpha/1
  Demux1/2 -> alpha/2
  Demux1/3 -> alpha/3
  Demux1/4 -> alpha/4
  calculatie alpha/1(alpha) -> MATLAB Function3/1(alpha), MATLAB Function2/4(alpha), MATLAB Function1/3(alpha), Display2/1, Demux1/1

== system ame532Project1_GimbalDynamicsModel_2023a/IMU  Aircraft dynamic sim1/mass & aero property calculation ==
  u : Inport
  CG calculation : MATLAB Function  TreatAsAtomicUnit=on
  Display : Display
  Display1 : Display
  J matrix : Display
  MATLAB Function : MATLAB Function  TreatAsAtomicUnit=on
  MATLAB Function1 : MATLAB Function  TreatAsAtomicUnit=on
  MATLAB Function2 : MATLAB Function  TreatAsAtomicUnit=on
  Mux : Mux  Inputs=3
  Submatrix : matrix_library/Submatrix  RowSpan=All rows  RowStartMode=First  RowStartIndex=1  RowEndMode=Last  RowEndIndex=1  ColSpan=One column  ColStartMode=First  ColStartIndex=1  ColEndMode=Last  ColEndIndex=1
  Sum of Elements : Sum  Inputs=+
  aero prop matrix x y z c b A AR : Display
  m matrix : Display
  x_b_sb : Display
  total mass : Outport
  cg coordinate : Outport  Port=2
  J_matrix : Outport  Port=3
  aero surface property matrix : Outport  Port=4
  x b sb : Outport  Port=5
  wires:
  CG calculation/1(cg_x) -> Mux/1
  u/1 -> MATLAB Function1/2(m_matrix), MATLAB Function2/1(M_matrix), m matrix/1, Submatrix/1, MATLAB Function/2(M_matrix), CG calculation/1(M_matrix)
  CG calculation/2(cg_y) -> Mux/2
  CG calculation/3(cg_z) -> Mux/3
  Mux/1 -> MATLAB Function1/3(cg_location), MATLAB Function/1(cg_location), cg coordinate/1, Display/1
  Submatrix/1 -> Sum of Elements/1
  Sum of Elements/1 -> total mass/1, Display1/1
  MATLAB Function/1(J_matrix) -> J_matrix/1, J matrix/1
  MATLAB Function2/1(aero_prop) -> MATLAB Function1/1(aero_prop_matrix), aero prop matrix x y z c b A AR/1, aero surface property matrix/1
  MATLAB Function1/1(x_b_s_ac) -> x b sb/1, x_b_sb/1

== system ame532Project1_GimbalDynamicsModel_2023a/IMU  Aircraft dynamic sim1/measurement subsystem ==
  velocity in body frame : Inport
  Asin : Trigonometry  Operator=asin
  Atan2 : Trigonometry  Operator=atan2
  Demux : Demux  Outputs=3
  Demux1 : Demux  Outputs=3
  Display : Display
  Divide : Product  Inputs=*/  RndMeth=Zero  SaturateOnIntegerOverflow=on
  MATLAB Function : MATLAB Function  TreatAsAtomicUnit=on
  Mux : Mux  Inputs=3
  Radians to Degrees{,1..3} (4 alike) : simulink_extras/Transformations/Radians to Degrees
  v_inf alpha beta : Scope  NumInputPorts=3
  total speed : Outport
  alpha (AoA) : Outport  Port=2
  beta (side slip) : Outport  Port=3
  wires:
  MATLAB Function/1(magnitude) -> Divide/2, Mux/1, total speed/1, v_inf alpha beta/1
  velocity in body frame/1 -> MATLAB Function/1(velocity), Demux1/1, Demux/1
  Demux/3 -> Atan2/1
  Demux/1 -> Atan2/2
  Atan2/1 -> alpha (AoA)/1, Radians to Degrees2/1, Radians to Degrees/1
  Demux1/2 -> Divide/1
  Divide/1 -> Asin/1
  Asin/1 -> beta (side slip)/1, Radians to Degrees3/1, Radians to Degrees1/1
  Mux/1 -> Display/1
  Radians to Degrees/1 -> Mux/2
  Radians to Degrees1/1 -> Mux/3
  Radians to Degrees2/1 -> v_inf alpha beta/2
  Radians to Degrees3/1 -> v_inf alpha beta/3

== system ame532Project1_GimbalDynamicsModel_2023a/IMU  Aircraft dynamic sim1/rotational dynamics ==
  note: body rate acceleration
  J_matrix : Inport
  Initial w : Inport  Port=2
  moment in body : Inport  Port=3
  Cross Product : matrix_library/Cross Product
  Display4 : Display
  Display5 : Display
  Display6 : Display
  Invert 3x3 Matrix : aerolibutil/Invert  3x3 Matrix
  Matrix Multiply4 : Product  Multiplication=Matrix(*)
  Matrix Multiply5 : Product  Multiplication=Matrix(*)
  Sum : Sum  Inputs=|+-
  body rate : Integrator  InitialConditionSource=external  InitialCondition=[0 0 0]'
  omega_b : Outport
  wires:
  Cross Product/1 -> Sum/2, Display6/1
  Sum/1 -> Matrix Multiply4/2
  J_matrix/1 -> Matrix Multiply5/1, Invert 3x3 Matrix/1
  body rate/1 -> omega_b/1, Matrix Multiply5/2, Cross Product/1
  Matrix Multiply4/1 -> Display5/1, body rate/1
  Invert 3x3 Matrix/1 -> Matrix Multiply4/1, Display4/1
  Matrix Multiply5/1 -> Cross Product/2
  Initial w/1 -> body rate/2
  moment in body/1 -> Sum/1

== system ame532Project1_GimbalDynamicsModel_2023a/IMU  Aircraft dynamic sim1/translational dynamics ==
  note: counter gravity before needs to be accounted by a DCM
  note: velocity in body frame
  note: acceleration in body frame
  p : Inport
  q : Inport  Port=2
  r : Inport  Port=3
  ZYXDCM : Inport  Port=4
  external forces : Inport  Port=5
  intial velocity : Inport  Port=6
  Display{,1..4,8..9} (7 alike) : Display
  Integrator5 : Integrator  InitialConditionSource=external
  MATLAB Function10 : MATLAB Function  TreatAsAtomicUnit=on
  Matrix Multiply6 : Product  Multiplication=Matrix(*)
  Matrix Multiply7 : Product  Multiplication=Matrix(*)
  Scope : Scope
  Sum : Sum  Inputs=|++-
  gravity in N_frame : Constant  Value=[0 0 9.81]'
  weight : Gain  Gain=1/0.48
  velocity in body frame : Outport
  wires:
  MATLAB Function10/1(Cross_Product_Matrix) -> Matrix Multiply7/1, Display8/1
  Integrator5/1 -> velocity in body frame/1, Display1/1, Matrix Multiply7/2
  Sum/1 -> Display3/1, Scope/1, Integrator5/1
  Matrix Multiply6/1 -> Sum/2, Display2/1
  Matrix Multiply7/1 -> Sum/3, Display9/1
  ZYXDCM/1 -> Display/1, Matrix Multiply6/1
  q/1 -> MATLAB Function10/2(q)
  p/1 -> MATLAB Function10/1(p)
  r/1 -> MATLAB Function10/3(r)
  intial velocity/1 -> Integrator5/2
  gravity in N_frame/1 -> Matrix Multiply6/2
  external forces/1 -> weight/1
  weight/1 -> Sum/1, Display4/1

== system ame532Project1_GimbalDynamicsModel_2023a/Subsystem/Equations of Motion ==
  initial location lat long alt : Inport
  AccelToVel : Integrator  InitialConditionSource=external  InitialCondition=[50;0;0]  ContinuousStateAttributes='Velocity_UVW'
  Accelerometer : Subsystem
  Aero Forces and Moments : Subsystem
  Degrees to Radians2 : simulink_extras/Transformations/Degrees to Radians
  Demux1 : Demux  Outputs=3
  Demux2 : Demux  Outputs=3
  Gyroscope : Subsystem
  Initial Body Velocity : Constant  Value=[13; 0; 0]
  Initial body rate : Constant  Value=[0 0 0]'
  Integrator : Integrator  InitialConditionSource=external
  LLA to ECEF Position : LLA2ECEF  ptype=Custom  R=earthRadius
  Manual Switch : ManualSwitch
  Manual Switch2 : ManualSwitch
  Mux6 : Mux  Inputs=2
  Rotational Dynamics : Subsystem
  Rotational Kinematics_Euler : Subsystem
  Rotational Kinematics_Quaternions : Subsystem  Commented=on
  Rotational Kinematics_Strapdown : Subsystem  Commented=on
  Scope{,1..3} (4 alike) : Scope
  Translational Dynamics : Subsystem
  Translational Kinematics : Subsystem
  c_B_N : MATLAB Function  TreatAsAtomicUnit=on
  Out Positon E_x_B_E_E : Outport
  position in LAX NED : Outport  Port=2
  DCM C_EB : Outport  Port=3
  wires:
  Translational Kinematics/1(E_x_B_E_E) -> Out Positon E_x_B_E_E/1
  initial location lat long alt/1 -> Demux1/1
  Demux1/1 -> Mux6/1
  Demux1/3 -> LLA to ECEF Position/2
  Mux6/1 -> LLA to ECEF Position/1
  Demux1/2 -> Mux6/2
  LLA to ECEF Position/1 -> Translational Kinematics/3(LAX Initial Loc)
  Rotational Dynamics/1(wdotVector Body Rates_PQR) -> Integrator/1  "wdotVector Body Rates_PQR"
  Initial body rate/1 -> Degrees to Radians2/1
  Degrees to Radians2/1 -> Integrator/2
  Aero Forces and Moments/1(Mext_B) -> Rotational Dynamics/2(Aero Moment)
  Aero Forces and Moments/2(Fext_B) -> Translational Dynamics/3(Aero Forces)
  Initial Body Velocity/1 -> AccelToVel/2
  AccelToVel/1 -> Translational Kinematics/1(Computed V_B_E_B), Scope1/1, Translational Dynamics/4(V_B_E_B), Aero Forces and Moments/1(V_B_E_B)
  Rotational Kinematics_Euler/1(Theta Vector_rad) -> Demux2/1  "Computed Attitude w.r.t ECEF"
  Demux2/1 -> c_B_N/3(roll_rad)
  Demux2/2 -> c_B_N/2(pitch_rad)
  Demux2/3 -> c_B_N/1(yaw_rad)
  c_B_N/1(outDCM) -> Translational Dynamics/1(C_B_N), Translational Kinematics/2(C_B_N), Aero Forces and Moments/2(C_B_N)  "c_B_N"
  Translational Kinematics/2(Out_C_E_B) -> DCM C_EB/1
  Translational Kinematics/3(Position LAX w.r.t NED) -> position in LAX NED/1
  Translational Dynamics/1(Out_Vdot_B_E_B) -> Accelerometer/1(True Acceleration), Manual Switch/2  "Vdot_B_E_B  Acceleration of Body w.r.t ECEF measured in Body"
  Accelerometer/1(Measured Acceleration) -> Manual Switch/1, Scope/1  "measured Vdot_B_E_B"
  Manual Switch/1 -> AccelToVel/1
  Integrator/1 -> Manual Switch2/2, Gyroscope/1(True Body Rates), Scope3/1
  Gyroscope/1(Measured Body Rates) -> Manual Switch2/1  "Measured Body Rates"
  Manual Switch2/1 -> Scope2/1, Rotational Kinematics_Euler/1(wVectorBodyRates_PQR)

== system ame532Project1_GimbalDynamicsModel_2023a/Subsystem/Equations of Motion/Accelerometer ==
  True Acceleration : Inport
  Band-Limited White Noise : simulink/Sources/Band-Limited White Noise  Cov=[0.00000000000000001]  Ts=0.01  seed=[23341]
  Bias : Constant  Value=[0.0000000025 0.0000000025 0.0000000025]
  Constant : Constant  Value=[0 0 0]
  Manual Switch : ManualSwitch
  Scale Factor : Gain  Gain=0.00000001
  Scope : Scope
  Sum : Sum  Inputs=|++
  Sum1 : Sum  Inputs=|++
  Measured Acceleration : Outport
  wires:
  True Acceleration/1 -> Sum/1
  Bias/1 -> Manual Switch/1
  Sum/1 -> Scale Factor/1
  Scale Factor/1 -> Sum1/1
  Band-Limited White Noise/1 -> Sum1/2, Scope/1
  Sum1/1 -> Measured Acceleration/1
  Constant/1 -> Manual Switch/2
  Manual Switch/1 -> Sum/2

== system ame532Project1_GimbalDynamicsModel_2023a/Subsystem/Equations of Motion/Aero Forces and Moments ==
  V_B_E_B : Inport
  C_B_N : Inport  Port=2
  Constant : Constant  Value=0
  Constant1 : Constant  Value=0
  Constant2 : Constant  Value=0
  F&M Horiz Stab Surface (S2) : Subsystem
  F&M Horiz Stab Surface (S3) : Subsystem
  F&M Right Wing and Servo Surface (S4) : Subsystem
  F&M Right Wing and Servo Surface (S5) : Subsystem
  Manual Switch : ManualSwitch  CurrentSetting=0
  Matrix Multiply : Product  Multiplication=Matrix(*)
  Mux5 : Mux  Inputs=3
  Scope : Scope
  Step : Step  Time=20  After=0  SampleTime=0
  Sum : Sum  Inputs=|+-
  Sum1 : Sum  Inputs=|++++
  Sum2 : Sum  Inputs=|++++
  Velocity of Air Mass w.r.t NED as Measured in NED : Constant  Value=[7 0 0]'
  Mext_B : Outport
  Fext_B : Outport  Port=2
  wires:
  V_B_E_B/1 -> Scope/1, F&M Right Wing and Servo Surface (S5)/1(v_B_E_B), F&M Right Wing and Servo Surface (S4)/1(v_B_E_B), F&M Horiz Stab Surface (S2)/1(v_B_E_B), F&M Horiz Stab Surface (S3)/1(v_B_E_B), Sum/1
  Velocity of Air Mass w.r.t NED as Measured in NED/1 -> Manual Switch/1  "V_A_N_N"
  Sum/1 -> F&M Horiz Stab Surface (S2)/2(V_B_A_B (Relative AIr Speed)), F&M Horiz Stab Surface (S3)/2(V_B_A_B (Relative AIr Speed)), F&M Right Wing and Servo Surface (S5)/2(V_B_A_B (Relative AIr Speed)), F&M Right Wing and Servo Surface (S4)/2(V_B_A_B (Relative AIr Speed))  "V_B_A_B (Relative AIr Speed)"
  F&M Horiz Stab Surface (S2)/2(LiftAndDragForceS2_B) -> Sum1/1
  F&M Horiz Stab Surface (S3)/2(LiftAndDragForceS3_B) -> Sum1/2
  F&M Right Wing and Servo Surface (S4)/2(LiftAndDragForceS4_B) -> Sum1/3
  F&M Right Wing and Servo Surface (S5)/2(LiftAndDragForceS5_B) -> Sum1/4
  Sum1/1 -> Fext_B/1
  F&M Horiz Stab Surface (S2)/1(momS2_B) -> Sum2/1
  F&M Horiz Stab Surface (S3)/1(momS3_B) -> Sum2/2
  F&M Right Wing and Servo Surface (S4)/1(momS4_B) -> Sum2/3
  F&M Right Wing and Servo Surface (S5)/1(momS5_B) -> Sum2/4
  Sum2/1 -> Mext_B/1
  C_B_N/1 -> Matrix Multiply/1
  Matrix Multiply/1 -> Sum/2  "V_A_N_B"
  Step/1 -> Mux5/1
  Constant2/1 -> Mux5/3
  Constant1/1 -> Mux5/2
  Mux5/1 -> Manual Switch/2
  Manual Switch/1 -> Matrix Multiply/2
  Constant/1 -> F&M Right Wing and Servo Surface (S5)/3(LeftAileronControl), F&M Right Wing and Servo Surface (S4)/3(RightAileronControl), F&M Horiz Stab Surface (S3)/3(RudderControl), F&M Horiz Stab Surface (S2)/3(ElevatorControl)

== system ame532Project1_GimbalDynamicsModel_2023a/Subsystem/Equations of Motion/Gyroscope ==
  True Body Rates : Inport
  Band-Limited White Noise : simulink/Sources/Band-Limited White Noise  Cov=[0.00000000000000000000000001]  Ts=0.01  seed=[23341]
  Constant : Constant  Value=[0 0 0]
  Gyro Constant Bias : Constant  Value=[0.0000000025 0.0000000025 0.0000000025]
  Gyro Scale Factor : Gain  Gain=0.0000000001
  Manual Switch : ManualSwitch
  Sum : Sum  Inputs=|++
  Sum1 : Sum  Inputs=|++
  Measured Body Rates : Outport
  wires:
  True Body Rates/1 -> Sum/1
  Gyro Constant Bias/1 -> Manual Switch/1
  Sum/1 -> Gyro Scale Factor/1
  Gyro Scale Factor/1 -> Sum1/1
  Band-Limited White Noise/1 -> Sum1/2
  Sum1/1 -> Measured Body Rates/1
  Constant/1 -> Manual Switch/2
  Manual Switch/1 -> Sum/2

== system ame532Project1_GimbalDynamicsModel_2023a/Subsystem/Equations of Motion/Rotational Dynamics ==
  wVector Body Rates_PQR : Inport
  Aero Moment : Inport  Port=2
  Cross Product : matrix_library/Cross Product
  Invert 3x3 Matrix : aerolibutil/Invert  3x3 Matrix
  Jmat : sharedutil/Create 3x3 Matrix  aMode=aMode
      settings: LibrarySourceBlock=aerolibutil/Create 3x3 Matrix
  Jxx : Constant  Value=Jxx
  Jxy : Constant  Value=Jxy
  Jxz : Constant  Value=Jxz
  Jyx : Constant  Value=Jyx
  Jyy : Constant  Value=Jyy
  Jyz : Constant  Value=Jyz
  Jzx : Constant  Value=Jzx
  Jzy : Constant  Value=Jzy
  Jzz : Constant  Value=Jzz
  Manual Switch : ManualSwitch
  Manual Switch1 : ManualSwitch  CurrentSetting=0
  Manual Switch3 : ManualSwitch  CurrentSetting=0
  Matrix Multiply2 : Product  Multiplication=Matrix(*)
  MatrixMultiply : Product  Multiplication=Matrix(*)
  Pitch Body Moment : Constant  Value=MM
  Roll Body Moment : Constant  Value=LL
  Sum : Sum  Inputs=|+-
  Using Cross Product Matrix : Subsystem
  Using Cross Product Operator Only : Subsystem
  Vector Concatenate : Concatenate  NumInputs=3
  Yaw Body Moment : Constant  Value=NN
  wdotVector Body Rates_PQR : Outport
  wires:
  Using Cross Product Matrix/1(OmegaJw) -> Manual Switch1/1  "OmegaJw [3x1]"
  Sum/1 -> Matrix Multiply2/2
  Matrix Multiply2/1 -> wdotVector Body Rates_PQR/1
  Jxx/1 -> Jmat/1
  Jxy/1 -> Jmat/2
  Jxz/1 -> Jmat/3
  Jyx/1 -> Jmat/4
  Jyy/1 -> Jmat/5
  Jyz/1 -> Jmat/6
  Jzx/1 -> Jmat/7
  Jzy/1 -> Jmat/8
  Jzz/1 -> Jmat/9
  Invert 3x3 Matrix/1 -> Matrix Multiply2/1  "Jinv"
  Roll Body Moment/1 -> Vector Concatenate/1
  Pitch Body Moment/1 -> Vector Concatenate/2
  Yaw Body Moment/1 -> Vector Concatenate/3
  Vector Concatenate/1 -> Manual Switch/2  "Mext_B"
  Aero Moment/1 -> Manual Switch/1
  Manual Switch/1 -> Sum/1
  Using Cross Product Operator Only/1(OmegaJw) -> Manual Switch1/2
  Jmat/1 -> Invert 3x3 Matrix/1, Using Cross Product Operator Only/2(J Matrix), Using Cross Product Matrix/2(J Matrix), MatrixMultiply/1
  Cross Product/1 -> Manual Switch3/2
  Manual Switch1/1 -> Manual Switch3/1
  Manual Switch3/1 -> Sum/2
  wVector Body Rates_PQR/1 -> MatrixMultiply/2, Using Cross Product Matrix/1(wPQR), Cross Product/1, Using Cross Product Operator Only/1(wPQR)
  MatrixMultiply/1 -> Cross Product/2

== system ame532Project1_GimbalDynamicsModel_2023a/Subsystem/Equations of Motion/Rotational Kinematics_Euler ==
  wVectorBodyRates_PQR : Inport
  Demux : Demux  Outputs=3
  EulerAngles : Integrator  InitialConditionSource=external  InitialCondition=[0;30;30]  ContinuousStateAttributes='EulerAngles_PhiThetaPsi'
  HinvMatrix : MATLAB Function  TreatAsAtomicUnit=on
  Initial Attitude_rad w.r.t ECEF : Constant  Value=[0; 0; 0]
  MatrixMultiply : Product  Multiplication=Matrix(*)
  Scope : Scope
  Terminator : Terminator
  Theta Vector_rad : Outport
  wires:
  HinvMatrix/1(hinv) -> MatrixMultiply/1
  MatrixMultiply/1 -> EulerAngles/1  "Theta Vector Dot"
  EulerAngles/1 -> Demux/1, Theta Vector_rad/1, Scope/1  "Theta Vector_rad"
  Demux/1 -> HinvMatrix/2(rollPhi)  "roll_rad"
  Demux/2 -> HinvMatrix/1(pitchTheta)  "pitch_rad"
  Demux/3 -> Terminator/1  "yaw_rad"
  wVectorBodyRates_PQR/1 -> MatrixMultiply/2  "wVector Body Rates_PQR"
  Initial Attitude_rad w.r.t ECEF/1 -> EulerAngles/2
